simulink model "ben_is_ben_ext"  (Simulink 7.9)
settings: Solver=FixedStepDiscrete  StartTime=0.0  StopTime=inf  RelTol=1e-3
settings Model: Creator=bas  LastModifiedBy=bas  SimulationMode=external
settings OptimizationCC: OptimizeModelRefInitCode=on  LifeSpan=1
settings HardwareCC: ProdEndianess=LittleEndian  ProdHWDeviceType=Generic->32-bit Embedded Processor
settings RTWCC: SystemTargetFile=nanonote.tlc  TemplateMakefile=nanonote.tmf  Description=Ben NanoNote  GenerateReport=on  ProcessScript=nanonote_make_rtw_hook  IncludeHyperlinkInReport=on  GenerateTraceInfo=on  GenerateTraceReport=on  GenerateTraceReportSl=on  GenerateTraceReportSf=on  GenerateTraceReportEml=on
settings CodeAppCC: IgnoreCustomStorageClasses=off
settings STFCustomTargetCC: CodeReplacementLibrary=ANSI_C  GenerateSampleERTMain=on  CombineOutputUpdateFcns=on  ERTCustomFileBanners=on  SupportContinuousTime=off  SupportNonInlinedSFcns=off  GRTInterface=off  SystemTargetFile=nanonote.tlc
settings ERTTargetCC: CodeReplacementLibrary=ANSI_C  MultiwordLength=2048  GenerateSampleERTMain=on  ParMdlRefBuildCompliant=off  CompOptLevelCompliant=off  ConcurrentExecutionCompliant=off  ERTFirstTimeCompliant=off  ModelStepFunctionPrototypeControlCompliant=off  CPPClassGenCompliant=off  ExtMode=on  ExtModeStaticAlloc=on  ExtModeMexArgs='ben' 0  InlinedParameterPlacement=NonHierarchical  ERTCustomFileTemplate=example_file_process.tlc  ConvertIfToSwitch=off  SuppressUnreachableDefaultCases=off
settings CustomProperty: Value=on

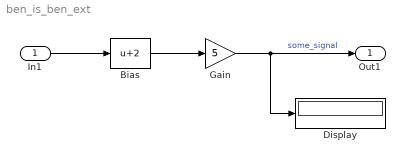
== system ben_is_ben_ext ==
  In1 : Inport
  Bias : Bias  Bias=2
  Display : Display
  Gain : Gain  Gain=5
  Out1 : Outport
  wires:
  In1/1 -> Bias/1
  Gain/1 -> Out1/1, Display/1  "some_signal"
  Bias/1 -> Gain/1
